simulink model "Sim1MPC"  (R2021b)
settings: Solver=VariableStepAuto  StartTime=0.0  StopTime=86400  RelTol=1e-3
settings Model: Creator=Rasoul  LastModifiedBy=Rasoul

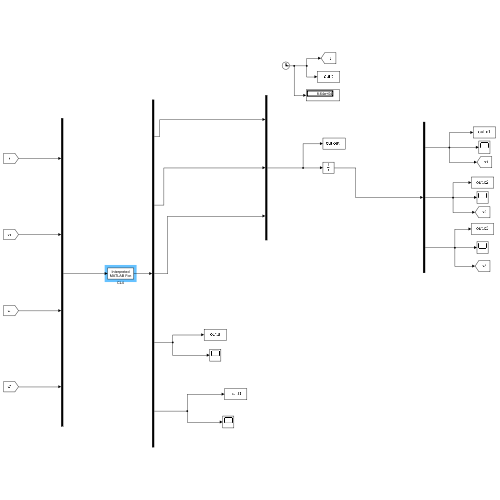
[thumbnail: Simulink's stored preview of the top-level diagram]
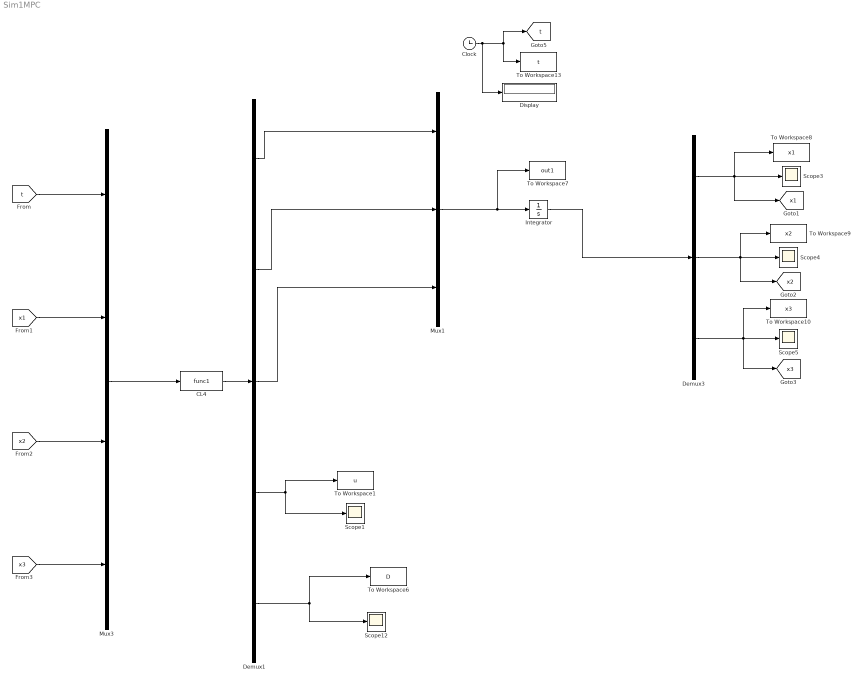
== system Sim1MPC ==
  CL4 : MATLABFcn  MATLABFcn=func1  OutputDimensions=5
  Clock : Clock
  Demux1 : Demux  Outputs=5
  Demux3 : Demux  Outputs=3
  Display : Display
  Integrator : Integrator  InitialCondition=[200;0;100]
  Mux1 : Mux  Inputs=3
  Mux3 : Mux
  Scope{1,3..5,12} (5 alike) : Scope
  To Workspace1 : ToWorkspace  VariableName=u  SampleTime=10
      settings: Save2DSignal=2-D array (concatenate along first dimension)
  To Workspace10 : ToWorkspace  VariableName=x3  SampleTime=10
      settings: Save2DSignal=2-D array (concatenate along first dimension)
  To Workspace13 : ToWorkspace  VariableName=t  SampleTime=10
      settings: Save2DSignal=2-D array (concatenate along first dimension)
  To Workspace6 : ToWorkspace  VariableName=D  SampleTime=10
      settings: Save2DSignal=2-D array (concatenate along first dimension)
  To Workspace7 : ToWorkspace  VariableName=out1  SampleTime=-1
      settings: Save2DSignal=2-D array (concatenate along first dimension)
  To Workspace8 : ToWorkspace  VariableName=x1  SampleTime=10
      settings: Save2DSignal=2-D array (concatenate along first dimension)
  To Workspace9 : ToWorkspace  VariableName=x2  SampleTime=10
      settings: Save2DSignal=2-D array (concatenate along first dimension)
  tag scope: t=global, x1=global, x2=global, x3=global
  wires:
  Mux3/1 -> CL4/1
  Demux3/1 -> [x1], Scope3/1, To Workspace8/1
  Demux1/3 -> Mux1/3
  Demux1/4 -> To Workspace1/1, Scope1/1
  [x2] -> Mux3/3
  [x1] -> Mux3/2
  CL4/1 -> Demux1/1
  Demux1/5 -> To Workspace6/1, Scope12/1
  Demux3/2 -> [x2], Scope4/1, To Workspace9/1
  Integrator/1 -> Demux3/1
  Demux1/2 -> Mux1/2
  [x3] -> Mux3/4
  Demux3/3 -> [x3], Scope5/1, To Workspace10/1
  Demux1/1 -> Mux1/1
  [t] -> Mux3/1
  Clock/1 -> Display/1, [t], To Workspace13/1
  Mux1/1 -> To Workspace7/1, Integrator/1
